simulink subsystem "Effect_of_Earths_Rotation"  (R2024a)
settings: Solver=VariableStepAuto  StartTime=0.0  StopTime=10.0  RelTol=1e-3
undefined symbols (not defined in the file): w_E
settings Model: Creator=Andrew Radulovich  LastModifiedBy=thatf
settings ModelReferenceCC: EnableRefExpFcnMdlSchedulingChecks=on
settings RTWCC: GPUComputeCapability=3.5

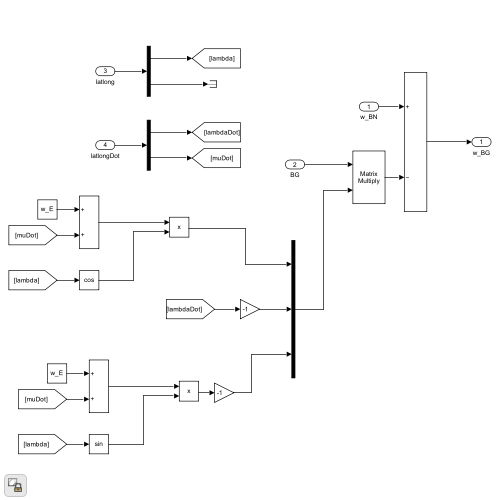
[thumbnail: Simulink's stored preview of the top-level diagram]
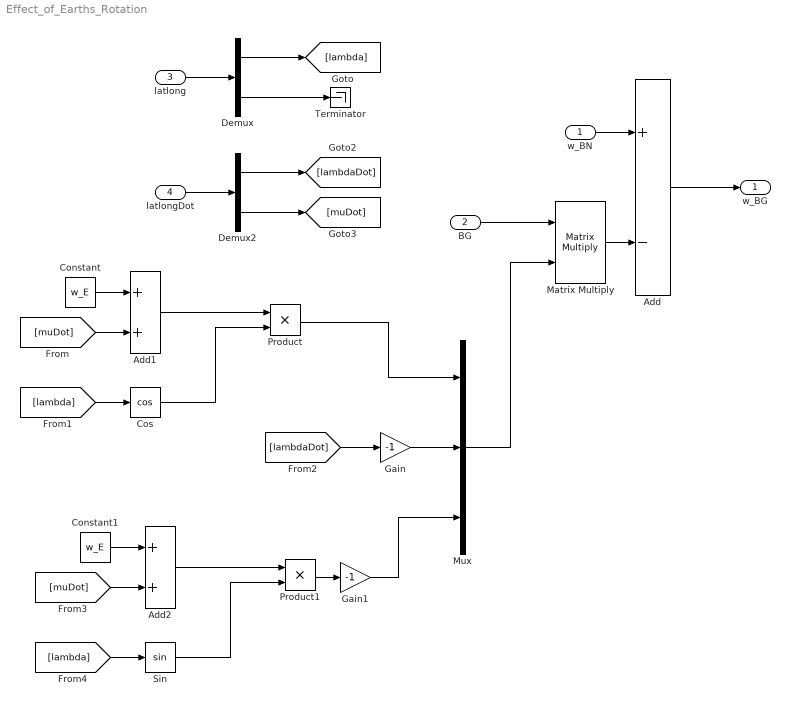
== system Effect_of_Earths_Rotation ==
  w_BN : Inport
  BG : Inport  Port=2
  latlong : Inport  Port=3
  latlongDot : Inport  Port=4
  Add : Sum  Inputs=+-
  Add1 : Sum
  Add2 : Sum
  Constant : Constant  Value=w_E
  Constant1 : Constant  Value=w_E
  Cos : Trigonometry  Operator=cos
  Demux : Demux  Outputs=2
  Demux2 : Demux  Outputs=2
  Gain : Gain  Gain=-1
  Gain1 : Gain  Gain=-1
  Matrix Multiply : Product  Multiplication=Matrix(*)
  Mux : Mux  Inputs=3
  Product : Product
  Product1 : Product
  Sin : Trigonometry
  Terminator : Terminator
  w_BG : Outport
  wires:
  Add/1 -> w_BG/1
  w_BN/1 -> Add/1
  Matrix Multiply/1 -> Add/2
  BG/1 -> Matrix Multiply/1
  Mux/1 -> Matrix Multiply/2
  latlong/1 -> Demux/1
  Demux/1 -> [lambda]
  Demux/2 -> Terminator/1
  latlongDot/1 -> Demux2/1
  Demux2/2 -> [muDot]
  Demux2/1 -> [lambdaDot]
  Constant/1 -> Add1/1
  [muDot] -> Add1/2
  Add1/1 -> Product/1
  Product/1 -> Mux/1
  Cos/1 -> Product/2
  [lambda] -> Cos/1
  [lambdaDot] -> Gain/1
  Gain/1 -> Mux/2
  Sin/1 -> Product1/2
  [lambda] -> Sin/1
  [muDot] -> Add2/2
  Add2/1 -> Product1/1
  Product1/1 -> Gain1/1
  Constant1/1 -> Add2/1
  Gain1/1 -> Mux/3
